simulink model "Heart_Insulin33"  (R2018a)
settings: Solver=VariableStepAuto  StartTime=0.0  StopTime=10.0  RelTol=1e-3
undefined symbols (not defined in the file): Q_i_B, Q_i_K, Q_i_L, Q_i_P, V_i_H, V_i_h
settings Model: Creator=cgonterman  LastModifiedBy=cgonterman

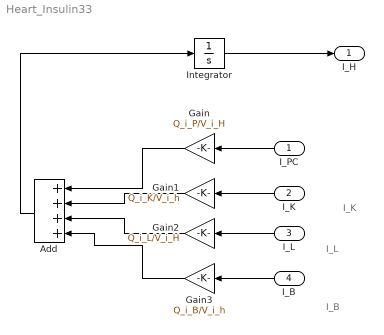
== system Heart_Insulin33 ==
  note: I_B
  note: I_L
  note: I_K
  "I_PC " : Inport
  "I_K " : Inport  Port=2
  "I_L " : Inport  Port=3
  "I_B " : Inport  Port=4
  Add : Sum  Inputs=++++
  Gain : Gain  Gain=Q_i_P/V_i_H
  Gain1 : Gain  Gain=Q_i_K/V_i_h
  Gain2 : Gain  Gain=Q_i_L/V_i_H
  Gain3 : Gain  Gain=Q_i_B/V_i_h
  Integrator : Integrator
  "I_H " : Outport
  wires:
  "I_PC "/1 -> Gain/1
  "I_K "/1 -> Gain1/1
  "I_L "/1 -> Gain2/1
  "I_B "/1 -> Gain3/1
  Gain/1 -> Add/1
  Gain1/1 -> Add/2
  Gain2/1 -> Add/3
  Gain3/1 -> Add/4
  Add/1 -> Integrator/1
  Integrator/1 -> "I_H "/1
